simulink model "game"  (R2022a)
settings: Solver=VariableStepAuto  StartTime=0.0  StopTime=Inf  RelTol=1e-3
libraries: robotlib x9
settings Model: Creator=michaelnaps  LastModifiedBy=sokajima
settings ModelReferenceCC: EnableRefExpFcnMdlSchedulingChecks=off
settings RTWCC: Description=Generic Real-Time Target

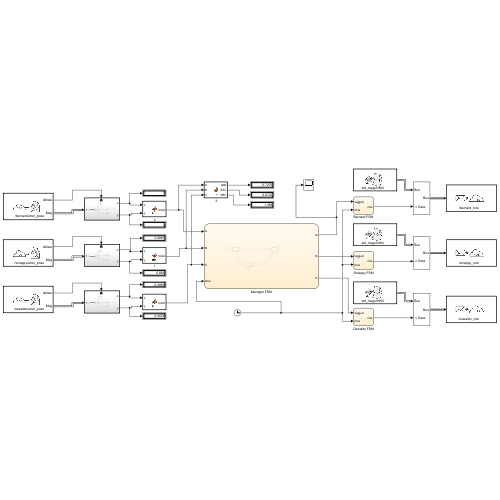
[thumbnail: Simulink's stored preview of the top-level diagram]
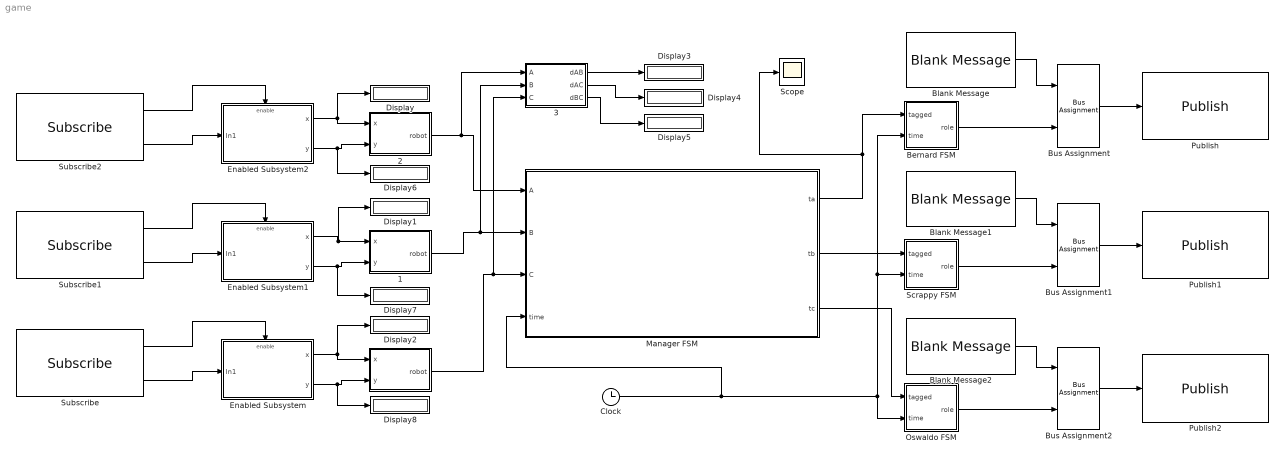
== system game ==
  " " : MATLAB Function  TreatAsAtomicUnit=on
  " 1" : MATLAB Function  TreatAsAtomicUnit=on
  " 2" : MATLAB Function  TreatAsAtomicUnit=on
  " 3" : MATLAB Function  TreatAsAtomicUnit=on
  Bernard FSM : Stateflow chart  TreatAsAtomicUnit=on
  Blank Message : robotlib/Blank Message  messageClass=Message  entityType=std_msgs/Int64  messageType=std_msgs/Int64  SampleTime=inf  legacyBusStruct=off
  Blank Message1 : robotlib/Blank Message  messageClass=Message  entityType=std_msgs/Int64  messageType=std_msgs/Int64  SampleTime=inf  legacyBusStruct=off
  Blank Message2 : robotlib/Blank Message  messageClass=Message  entityType=std_msgs/Int64  messageType=std_msgs/Int64  SampleTime=inf  legacyBusStruct=off
  Bus Assignment : BusAssignment  AssignedSignals=Data
  Bus Assignment1 : BusAssignment  AssignedSignals=Data
  Bus Assignment2 : BusAssignment  AssignedSignals=Data
  Clock : Clock
  Display{,1..8} (9 alike) : Display
  Enabled Subsystem : Subsystem
  Enabled Subsystem1 : Subsystem
  Enabled Subsystem2 : Subsystem
  Manager FSM : Stateflow chart  TreatAsAtomicUnit=on
  Oswaldo FSM : Stateflow chart  TreatAsAtomicUnit=on
  Publish : robotlib/Publish  topicSource=Specify your own  topic=/bernard_role  messageType=std_msgs/Int64  legacyBusStruct=off  messageQueueLength=10
  Publish1 : robotlib/Publish  topicSource=Specify your own  topic=/scrappy_role  messageType=std_msgs/Int64  legacyBusStruct=off  messageQueueLength=10
  Publish2 : robotlib/Publish  topicSource=Specify your own  topic=/oswaldo_role  messageType=std_msgs/Int64  legacyBusStruct=off  messageQueueLength=10
  Scope : Scope
  Scrappy FSM : Stateflow chart  TreatAsAtomicUnit=on
  Subscribe : robotlib/Subscribe  topicSource=Specify your own  topic=/oswaldo/amcl_pose  messageType=geometry_msgs/PoseWithCovarianceStamped  SampleTime=0.03  legacyBusStruct=off  messageQueueLength=1
  Subscribe1 : robotlib/Subscribe  topicSource=Specify your own  topic=/scrappy/amcl_pose  messageType=geometry_msgs/PoseWithCovarianceStamped  SampleTime=0.03  legacyBusStruct=off  messageQueueLength=1
  Subscribe2 : robotlib/Subscribe  topicSource=Specify your own  topic=/bernard/amcl_pose  messageType=geometry_msgs/PoseWithCovarianceStamped  SampleTime=0.03  legacyBusStruct=off  messageQueueLength=1
  wires:
  Manager FSM/1(ta) -> Scope/1, Bernard FSM/1(tagged)
  Manager FSM/3(tc) -> Oswaldo FSM/1(tagged)
  Manager FSM/2(tb) -> Scrappy FSM/1(tagged)
  Clock/1 -> Manager FSM/4(time), Bernard FSM/2(time), Scrappy FSM/2(time), Oswaldo FSM/2(time)
  Subscribe/1 -> Enabled Subsystem/Enable
  Subscribe/2 -> Enabled Subsystem/1(In1)
  Enabled Subsystem/1(x) -> Display2/1, " "/1(x)
  Enabled Subsystem/2(y) -> Display8/1, " "/2(y)
  Enabled Subsystem1/1(x) -> Display1/1, " 1"/1(x)
  Enabled Subsystem1/2(y) -> Display7/1, " 1"/2(y)
  Subscribe1/2 -> Enabled Subsystem1/1(In1)
  Subscribe1/1 -> Enabled Subsystem1/Enable
  Enabled Subsystem2/1(x) -> Display/1, " 2"/1(x)
  Enabled Subsystem2/2(y) -> Display6/1, " 2"/2(y)
  Subscribe2/2 -> Enabled Subsystem2/1(In1)
  Subscribe2/1 -> Enabled Subsystem2/Enable
  " 2"/1(robot) -> " 3"/1(A), Manager FSM/1(A)
  " 1"/1(robot) -> " 3"/2(B), Manager FSM/2(B)
  " "/1(robot) -> " 3"/3(C), Manager FSM/3(C)
  Blank Message/1 -> Bus Assignment/1
  Bernard FSM/1(role) -> Bus Assignment/2
  Bus Assignment/1 -> Publish/1
  Blank Message1/1 -> Bus Assignment1/1
  Blank Message2/1 -> Bus Assignment2/1
  Oswaldo FSM/1(role) -> Bus Assignment2/2
  Bus Assignment2/1 -> Publish2/1
  Bus Assignment1/1 -> Publish1/1
  Scrappy FSM/1(role) -> Bus Assignment1/2
  " 3"/1(dAB) -> Display3/1
  " 3"/2(dAC) -> Display4/1
  " 3"/3(dBC) -> Display5/1

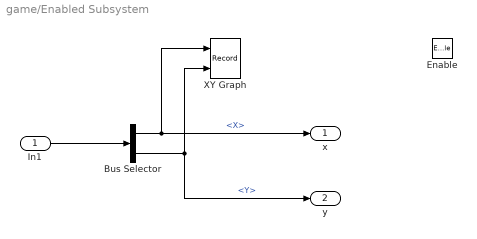
== system game/Enabled Subsystem ==
  In1 : Inport
  Enable : EnablePort
  Bus Selector : BusSelector  DialogController=Simulink.DDGSource_BusSelector  OutputSignals=Pose.Pose.Position.X,Pose.Pose.Position.Y
  XY Graph : Record  FileSettingsInternal="{\"entries\":[{\"content\":{\"excelSettings\":{\"content\":{},\"type\":\"Streamout.ExcelSettings\"}},\"type\":\"Streamout.FileSettingStorage\",\"uuid\":\"f427c31b-d706-4241-ad94-a47137b0d2c9\"}],\"packageUris\":[\"http://schema.mathworks.com/mf0/streamout_blocks/R2020a\"],\"version\":\"1.0\"}"  Layout=[1 1]  SignalsInternal="{\"entries\":[{\"content\":{\"signals\":[{\"content\":{\"blockPath\":[\"game2022a/Enabled Subsystem/XY Graph\"],\"channel\":[],\"dimensions\":[1],\"domain\":\"game2022a/Enabled Subsystem/XY Graph\",\"lineColor\":\"#a2142f\",\"plots\":[1],\"port\":1,\"sid\":[\"\"],\"signalID\":6826,\"signalName\":\"<X>\"},\"type\":\"RecordBlkView.Signal\",\"uuid\":\"641d6e73-6168-4ff5-ba53-9002d22d5f9e\"},{\"content\":{\"blockPath\":[\"game2022a/Enabled Subsystem/XY Graph\"],\"channel\":[],\"dimensions\":[1],\"domain\":\"game2022a/Enabled Subsystem/XY Graph\",\"lineColor\":\"#139fff\",\"plots\":[1],\"port\":2,\"sid\":[\"\"],\"signalID\":6830,\"signalName\":\"<Y>\"},\"type\":\"RecordBlkView.Signal\",\"uuid\":\"4f889dea-b4eb-4b73-a80d-9716052a6940\"}]},\"type\":\"RecordBlkView.InputSignals\",\"uuid\":\"62dd2a83-ddb6-401b-b59e-d04de35e801b\"}],\"packageUris\":[\"http://schema.mathworks.com/mf0/streamout_blocks/R2020a\"],\"version\":\"1.0\"}"  VisualizationBindings="{\"xyplotplugin\":{\"info\":[{\"series\":[{\"bindingParametersList\":[{\"parameter\":\"X-Axis\",\"signalID\":6826,\"signalName\":\"<X>\"},{\"parameter\":\"Y-Axis\",\"signalID\":6830,\"signalName\":\"<Y>\"}],\"seriesID\":34839}],\"subplotID\":1}]}}"  CompatibilityTag=XY  st=-1
  x : Outport  VectorParamsAs1DForOutWhenUnconnected=off
  y : Outport  Port=2  VectorParamsAs1DForOutWhenUnconnected=off
  wires:
  In1/1 -> Bus Selector/1
  Bus Selector/2 -> y/1, XY Graph/2  "<Y>"
  Bus Selector/1 -> x/1, XY Graph/1  "<X>"

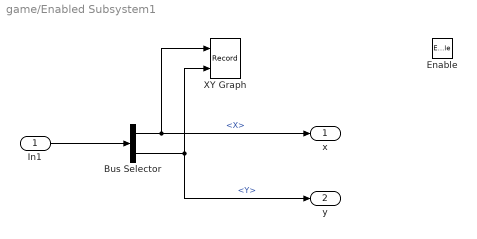
== system game/Enabled Subsystem1 ==
  In1 : Inport
  Enable : EnablePort
  Bus Selector : BusSelector  DialogController=Simulink.DDGSource_BusSelector  OutputSignals=Pose.Pose.Position.X,Pose.Pose.Position.Y
  XY Graph : Record  FileSettingsInternal="{\"entries\":[{\"content\":{\"excelSettings\":{\"content\":{},\"type\":\"Streamout.ExcelSettings\"}},\"type\":\"Streamout.FileSettingStorage\",\"uuid\":\"67ba3dff-513c-402a-9726-0bbd28852940\"}],\"packageUris\":[\"http://schema.mathworks.com/mf0/streamout_blocks/R2020a\"],\"version\":\"1.0\"}"  Layout=[1 1]  SignalsInternal="{\"entries\":[{\"content\":{\"signals\":[{\"content\":{\"blockPath\":[\"game2022a/Enabled Subsystem1/XY Graph\"],\"channel\":[],\"dimensions\":[1],\"domain\":\"game2022a/Enabled Subsystem1/XY Graph\",\"lineColor\":\"#a2142f\",\"plots\":[1],\"port\":1,\"sid\":[\"\"],\"signalID\":6818,\"signalName\":\"<X>\"},\"type\":\"RecordBlkView.Signal\",\"uuid\":\"12ee7c0e-da2c-4a70-b8ea-47a7a77d3b1f\"},{\"content\":{\"blockPath\":[\"game2022a/Enabled Subsystem1/XY Graph\"],\"channel\":[],\"dimensions\":[1],\"domain\":\"game2022a/Enabled Subsystem1/XY Graph\",\"lineColor\":\"#139fff\",\"plots\":[1],\"port\":2,\"sid\":[\"\"],\"signalID\":6822,\"signalName\":\"<Y>\"},\"type\":\"RecordBlkView.Signal\",\"uuid\":\"9fe79f4c-6a7a-40aa-abdf-6b5239301d46\"}]},\"type\":\"RecordBlkView.InputSignals\",\"uuid\":\"011b23fc-ca64-4bfb-bd22-e0d11e339817\"}],\"packageUris\":[\"http://schema.mathworks.com/mf0/streamout_blocks/R2020a\"],\"version\":\"1.0\"}"  VisualizationBindings="{\"xyplotplugin\":{\"info\":[{\"series\":[{\"bindingParametersList\":[{\"parameter\":\"X-Axis\",\"signalID\":6818,\"signalName\":\"<X>\"},{\"parameter\":\"Y-Axis\",\"signalID\":6822,\"signalName\":\"<Y>\"}],\"seriesID\":8827}],\"subplotID\":1}]}}"  CompatibilityTag=XY  st=-1
  x : Outport  VectorParamsAs1DForOutWhenUnconnected=off
  y : Outport  Port=2  VectorParamsAs1DForOutWhenUnconnected=off
  wires:
  In1/1 -> Bus Selector/1
  Bus Selector/2 -> y/1, XY Graph/2  "<Y>"
  Bus Selector/1 -> x/1, XY Graph/1  "<X>"

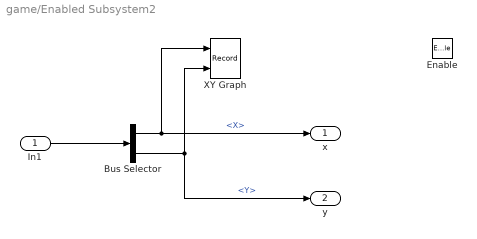
== system game/Enabled Subsystem2 ==
  In1 : Inport
  Enable : EnablePort
  Bus Selector : BusSelector  DialogController=Simulink.DDGSource_BusSelector  OutputSignals=Pose.Pose.Position.X,Pose.Pose.Position.Y
  XY Graph : Record  FileSettingsInternal="{\"entries\":[{\"content\":{\"excelSettings\":{\"content\":{},\"type\":\"Streamout.ExcelSettings\"}},\"type\":\"Streamout.FileSettingStorage\",\"uuid\":\"026d82cc-2f0f-4972-8cdd-d594e1a3bc60\"}],\"packageUris\":[\"http://schema.mathworks.com/mf0/streamout_blocks/R2020a\"],\"version\":\"1.0\"}"  Layout=[1 1]  SignalsInternal="{\"entries\":[{\"content\":{\"signals\":[{\"content\":{\"blockPath\":[\"game2022a/Enabled Subsystem2/XY Graph\"],\"channel\":[],\"dimensions\":[1],\"domain\":\"game2022a/Enabled Subsystem2/XY Graph\",\"lineColor\":\"#77ac30\",\"plots\":[],\"port\":1,\"sid\":[\"\"],\"signalID\":6810,\"signalName\":\"<X>\"},\"type\":\"RecordBlkView.Signal\",\"uuid\":\"54d8e471-38ca-4e91-b130-f51c04596ccf\"},{\"content\":{\"blockPath\":[\"game2022a/Enabled Subsystem2/XY Graph\"],\"channel\":[],\"dimensions\":[1],\"domain\":\"game2022a/Enabled Subsystem2/XY Graph\",\"lineColor\":\"#4dbeee\",\"plots\":[],\"port\":2,\"sid\":[\"\"],\"signalID\":6814,\"signalName\":\"<Y>\"},\"type\":\"RecordBlkView.Signal\",\"uuid\":\"5becf699-307c-4a06-a4af-c61ac29c344f\"}]},\"type\":\"RecordBlkView.InputSignals\",\"uuid\":\"f85e57cd-72e8-4678-baf0-03a8b908ce90\"}],\"packageUris\":[\"http://schema.mathworks.com/mf0/streamout_blocks/R2020a\"],\"version\":\"1.0\"}"  VisualizationBindings="{\"xyplotplugin\":{\"info\":[{\"series\":[],\"subplotID\":1}]}}"  CompatibilityTag=XY  st=-1
  x : Outport  VectorParamsAs1DForOutWhenUnconnected=off
  y : Outport  Port=2  VectorParamsAs1DForOutWhenUnconnected=off
  wires:
  In1/1 -> Bus Selector/1
  Bus Selector/2 -> y/1, XY Graph/2  "<Y>"
  Bus Selector/1 -> x/1, XY Graph/1  "<X>"

== stateflow chart game/Oswaldo FSM ==
  state S_pursuer
    %role = "pursuer"
    role = 1;
  state S_evader
    %role = "evader"
    role = 2;
  state S_delay
    %role = "paused"
    role = 3;
  (default) -> S_evader
  S_pursuer -> S_evader : [tagged]
  S_delay -> S_pursuer [order 1] : [(time - p_start) >= T]
  S_evader -> S_delay : [tagged]{p_start = time}
  S_delay -> S_delay [order 2] : [(time - p_start) < T]
  data: tagged input; role output; T constant double =5; p_start local; time input

== matlab function game/ 1 ==
  data: x input; robot output; y input
function robot = fcn(x,y)
    robot = [x, y];
end

== matlab function game/ 2 ==
  data: x input; robot output; y input
function robot = fcn(x,y)
    robot = [x, y];
end

== matlab function game/ 3 ==
  data: A input; dAB output; B input; C input; dAC output; dBC output
function [dAB, dAC, dBC] = fcn(A,B,C)
    dAB = distance_robot(A,B);
    dAC = distance_robot(A,C);
    dBC = distance_robot(B,C);
end

== stateflow chart game/Bernard FSM ==
  state S_pursuer
    %role = "pursuer"
    role = 1;
  state S_evader
    %role = "evader"
    role  =2;
  state S_delay
    %role = "paused"
    role = 3;
  (default) -> S_pursuer
  S_pursuer -> S_evader : [tagged]
  S_delay -> S_pursuer [order 1] : [(time - p_start) >= T]
  S_evader -> S_delay : [tagged]{p_start = time}
  S_delay -> S_delay [order 2] : [(time - p_start) < T]
  data: tagged input; role output; time input double =get_param(bdroot,'FixedStep'); T constant double =5; p_start local

== matlab function game/  ==
  data: x input; robot output; y input
function robot = fcn(x,y)
    robot = [x, y];
end

== stateflow chart game/Manager FSM ==
  state S_ABC
    %ta = 0;
    %tb = 0;
    %tc = 0;
  state S_BAC
    %ta = 0;
    %tb = 0;
    %tc = 0;
  state S_CAB
    %ta = 0;
    %tb = 0;
    %tc = 0;
  (default) -> S_ABC : {p_start = time}
  S_BAC -> S_BAC [order 3] : [distance_robot(A,B) > W && distance_robot(A,C) > W]{ta=0, tb=0, tc=0}
  S_ABC -> S_ABC [order 3] : [distance_robot(A,B) > W && distance_robot(A,C) > W]{ta=0, tb=0, tc=0;}
  S_ABC -> S_BAC [order 1] : [distance_robot(A,B) <= W && time - p_start >= T]{ta = 1, tb = 1, p_start = time}
  S_BAC -> S_ABC [order 2] : [distance_robot(B,A) <= W && time - p_start >= T]{ta = 1, tb = 1, p_start = time}
  S_ABC -> S_CAB [order 2] : [distance_robot(C,A) <= W && time - p_start >= T]{ta = 1, tc = 1, p_start = time}
  S_CAB -> S_ABC [order 2] : [distance_robot(C,A) <= W && time - p_start >= T]{ta = 1, tc = 1, p_start = time}
  S_CAB -> S_BAC [order 1] : [distance_robot(C,B) <= W && time - p_start >= T]{tb = 1, tc = 1, p_start = time}
  S_BAC -> S_CAB [order 1] : [distance_robot(B,C) <= W && time - p_start >= T]{tb = 1, tc = 1, p_start = time}
  S_CAB -> S_CAB [order 3] : [distance_robot(A,B) > W && distance_robot(A,C) > W]{ta=0, tb=0, tc=0}
  data: ta output; tb output; tc output; A input; B input; C input; W constant double =tag_radius; p_start local; time input; T constant double =5; a constant double; b constant double; c constant double; dist local

== stateflow chart game/Scrappy FSM ==
  state S_pursuer
    %role = "pursuer"
    role = 1;
  state S_evader
    %role = "evader"
    role = 2;
  state S_delay
    %role = "paused"
    role = 3;
  (default) -> S_evader
  S_pursuer -> S_evader : [tagged]
  S_delay -> S_pursuer [order 1] : [(time - p_start) >= T]
  S_evader -> S_delay : [tagged]{p_start = time}
  S_delay -> S_delay [order 2] : [(time - p_start) < T]
  data: tagged input; role output; T constant double =5; p_start local; time input
